simulink model "single_cell_battery"  (R2025b)
settings: Solver=FixedStepDiscrete  StartTime=0.0  StopTime=1400  FixedStep=0.1  RelTol=1e-3
values from neighbouring files (symbols this model uses):
  ocv_tbl = [3.00794729414 3.13855268975 3.26915808536 3.36367221502 3.42121073522 3.48509573231 3.53283075862 3.56520306642 3.59211861232 3.62170414448 3.65292960138 3.70049709897 ... (21 elements, 21x1)]    [params_all_temps_final.mat]
  Q_nom = 2.995    [params_10C_final.mat]    (also in params_all_temps_final.mat)
  soc_bp = [0 0.05 0.1 0.15 0.2 0.25 0.3 0.35 0.4 0.45 0.5 0.55 ... (21 elements, 21x1)]    [params_all_temps_final.mat]
  soc_common = [0.17 0.245454545455 0.320909090909 0.396363636364 0.471818181818 0.547272727273 0.622727272727 0.698181818182 0.773636363636 0.849090909091 0.924545454545 1]    [params_all_temps_final.mat]
  temp_bp = [0 10 25]    [params_all_temps_final.mat]
  Ts = 0.1    [params_10C_final.mat]    (also in params_all_temps_final.mat)
undefined symbols (not defined in the file or in its folder): C1, C2, DiscIntNeverNeededParam, I_test, inv_C1_2d_fixed, neg_inv_R1C1_2d_fixed, R0, R0_2d_fix, R1, R2, SoC_init
settings Model: PacingRate=0.890000  Creator=mahad  LastModifiedBy=mahad
settings DataIOCC: SignalLogging=off  SaveTime=off
settings DebuggingCC: ReadBeforeWriteMsg=DisableAll  WriteAfterWriteMsg=DisableAll  WriteAfterReadMsg=DisableAll  MultiTaskDSMMsg=none
settings ModelReferenceCC: UpdateModelReferenceTargets=IfOutOfDate
settings SFSimCC: SFSimEcho=off

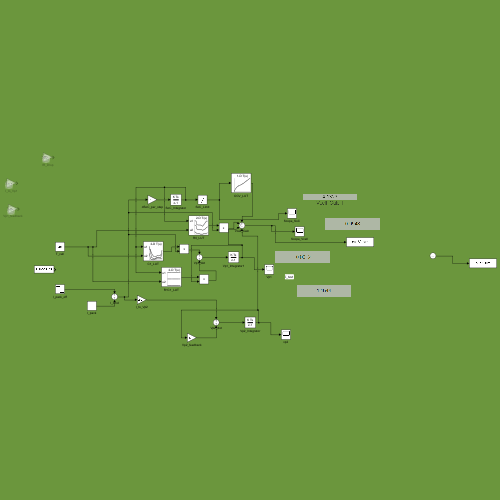
[thumbnail: Simulink's stored preview of the top-level diagram]
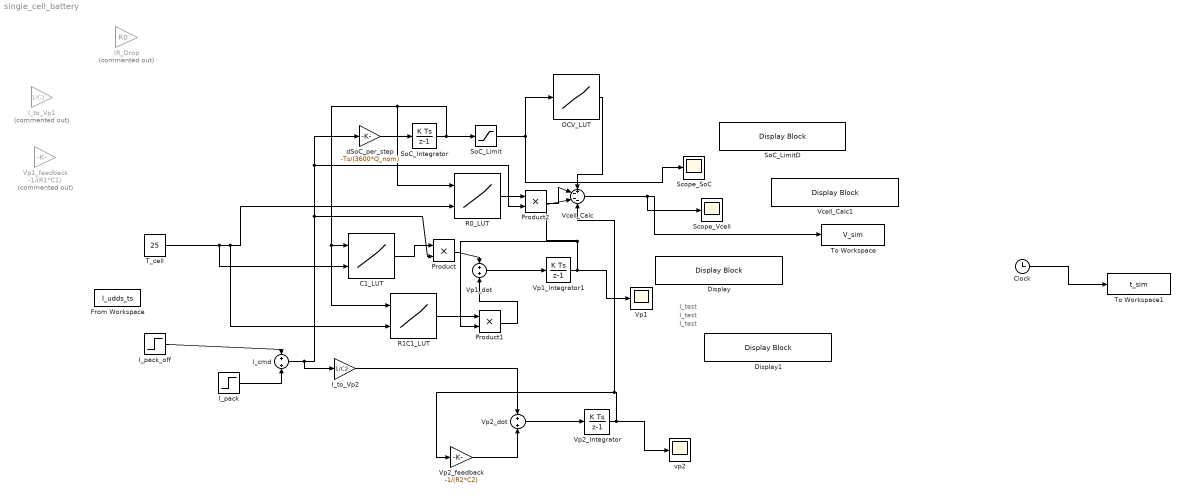
== system single_cell_battery ==
  note: I_test
  note: I_test
  note: I_test
  C1_LUT : Lookup_n-D  BreakpointsForDimension1=soc_common  BreakpointsForDimension2=temp_bp  Table=inv_C1_2d_fixed  ExtrapMethod=Clip  InternalRulePriority=Speed  RndMeth=Simplest
      settings: InputPortMap=u0,u1
  Clock : Clock
  Display : DisplayBlock  LabelPosition=Hide  Transparency=1  GridColor=[0.502, 0.502, 0.502]
  Display1 : DisplayBlock  LabelPosition=Hide  Transparency=1  GridColor=[0.502, 0.502, 0.502]
  From Workspace : FromWorkspace  VariableName=I_udds_ts
  IR_Drop : Gain  Commented=on  Gain=R0
  I_cmd : Sum
  I_pack : Step  Time=0  After=I_test  SampleTime=0.1
  I_pack_off : Step  Time=10  After=-I_test  SampleTime=0.1
  I_to_Vp1 : Gain  Commented=on  Gain=1/C1
  I_to_Vp2 : Gain  Gain=1/C2
  OCV_LUT : Lookup_n-D  NumberOfTableDimensions=1  BreakpointsForDimension1=soc_bp  BreakpointsForDimension2=[]  BeginIndexSearchUsingPreviousIndexResult=on  Table=ocv_tbl  ExtrapMethod=Clip  InternalRulePriority=Speed  RndMeth=Simplest
  Product : Product
  Product1 : Product
  Product2 : Product
  R0_LUT : Lookup_n-D  BreakpointsForDimension1=soc_common  BreakpointsForDimension2=temp_bp  Table=R0_2d_fix  ExtrapMethod=Clip  InternalRulePriority=Speed  RndMeth=Simplest
      settings: InputPortMap=u0,u1
  R1C1_LUT : Lookup_n-D  BreakpointsForDimension1=soc_common  BreakpointsForDimension2=temp_bp  Table=neg_inv_R1C1_2d_fixed  ExtrapMethod=Clip  InternalRulePriority=Speed  RndMeth=Simplest
      settings: InputPortMap=u0,u1
  Scope_SoC : Scope
      settings: ActiveDisplayYMinimum=-1  ActiveDisplayYMaximum=1  DataLoggingVariableName=SoC_log
  Scope_Vcell : Scope
      settings: ActiveDisplayYMinimum=3.9069471530318669  ActiveDisplayYMaximum=4.2003229383111682
  SoC_Integrator : DiscreteIntegrator  InitialCondition=SoC_init  SampleTime=0.1  ICPrevOutput=DiscIntNeverNeededParam  ICPrevScaledInput=DiscIntNeverNeededParam
  SoC_Limit : Saturate  UpperLimit=1  LowerLimit=0
  SoC_LimitD : DisplayBlock  LabelPosition=Bottom  Transparency=1  GridColor=[0.502, 0.502, 0.502]
  T_cell : Constant  Value=25
  To Workspace : ToWorkspace  VariableName=V_sim  SampleTime=-1
  To Workspace1 : ToWorkspace  VariableName=t_sim  SampleTime=-1
  Vcell_Calc : Sum  Inputs=+---
  Vcell_Calc1 : DisplayBlock  LabelPosition=Hide  Transparency=1  GridColor=[0.502, 0.502, 0.502]
  Vp1 : Scope
      settings: ActiveDisplayYMinimum=-0.0028893234136200406  ActiveDisplayYMaximum=0.026003910722580369  DataLoggingVariableName=ScopeData2
  Vp1_Integrator1 : DiscreteIntegrator  SampleTime=0.1  ICPrevOutput=DiscIntNeverNeededParam  ICPrevScaledInput=DiscIntNeverNeededParam
  Vp1_dot : Sum
  Vp1_feedback : Gain  Commented=on  Gain=-1/(R1*C1)
  Vp2_Integrator : DiscreteIntegrator  SampleTime=0.1  ICPrevOutput=DiscIntNeverNeededParam  ICPrevScaledInput=DiscIntNeverNeededParam
  Vp2_dot : Sum
  Vp2_feedback : Gain  Gain=-1/(R2*C2)
  dSoC_per_step : Gain  Gain=-Ts/(3600*Q_nom)
  vp2 : Scope
      settings: ActiveDisplayYMinimum=-0.00021306760205067724  ActiveDisplayYMaximum=0.0019176084184560956  DataLoggingVariableName=ScopeData3
  wires:
  dSoC_per_step/1 -> SoC_Integrator/1
  SoC_Integrator/1 -> R1C1_LUT/1, C1_LUT/1, R0_LUT/1, SoC_Limit/1
  SoC_Limit/1 -> OCV_LUT/1, Scope_SoC/1
  OCV_LUT/1 -> Vcell_Calc/1
  Vcell_Calc/1 -> To Workspace/1, Scope_Vcell/1
  Vp1_Integrator1/1 -> Vp1/1, Product1/2, Vcell_Calc/3
  Vp1_dot/1 -> Vp1_Integrator1/1
  Vp2_dot/1 -> Vp2_Integrator/1
  Vp2_Integrator/1 -> vp2/1, Vcell_Calc/4, Vp2_feedback/1
  I_to_Vp2/1 -> Vp2_dot/1
  Vp2_feedback/1 -> Vp2_dot/2
  I_cmd/1 -> I_to_Vp2/1, Product2/2, dSoC_per_step/1, Product/2
  Clock/1 -> To Workspace1/1
  C1_LUT/1 -> Product/1
  Product/1 -> Vp1_dot/1
  R1C1_LUT/1 -> Product1/1
  Product1/1 -> Vp1_dot/2
  T_cell/1 -> C1_LUT/2, R1C1_LUT/2, R0_LUT/2
  R0_LUT/1 -> Product2/1
  Product2/1 -> Vcell_Calc/2
  I_pack_off/1 -> I_cmd/1
  I_pack/1 -> I_cmd/2
